simulink model "PP_vs_LQ_controllers_sim"  (R2019b)
settings: Solver=FixedStepAuto  StartTime=0.0  StopTime=10.0  FixedStep=0.002  RelTol=1e-3
values from neighbouring files (symbols this model uses):
  Ao = A-L*C    [StabilizationControl.m]
  Bo = [B,L]    [StabilizationControl.m]
  Co = eye(4)    [StabilizationControl.m]
  Klqi_int = Klqi(5)    [StabilizationControl.m]
  Klqi_state = Klqi(1:4)    [StabilizationControl.m]
  Kpp_int = Kpp_i(5)    [StabilizationControl.m]
  Kpp_state = Kpp_i(1:4)    [StabilizationControl.m]
undefined symbols (not defined in the file or in its folder): kalmf, Parameters
settings Model: Creator=Samsung  LastModifiedBy=Samsung

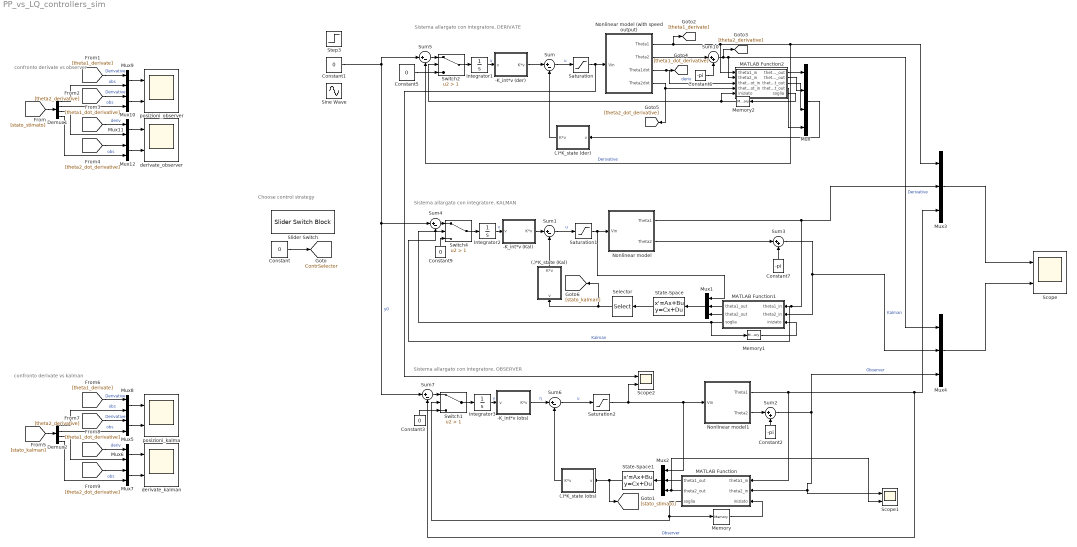
== system PP_vs_LQ_controllers_sim ==
  note: confronto derivate vs observer
  note: Choose control strategy
  note: Sistema allargato con integratore, DERIVATE
  note: Sistema allargato con integratore, KALMAN
  note: Sistema allargato con integratore, OBSERVER
  note: confronto derivate vs kalman
  (.)*K_state (Kal) : Subsystem
  "(.)*K_state (der) " : Subsystem
  (.)*K_state (obs) : Subsystem
  -K_int*v (Kal) : Subsystem
  -K_int*v (der) : Subsystem
  -K_int*v (obs) : Subsystem
  Constant{,1,3,5,9} (5 alike) : Constant  Value=0
  Constant2 : Constant  Value=-pi
  Constant6 : Constant  Value=-pi
  Constant7 : Constant  Value=-pi
  Demux1 : Demux
  Demux2 : Demux
  Integrator1 : Integrator
  Integrator2 : Integrator
  Integrator3 : Integrator
  MATLAB Function : MATLAB Function  TreatAsAtomicUnit=on
  MATLAB Function1 : MATLAB Function  TreatAsAtomicUnit=on
  MATLAB Function2 : MATLAB Function  TreatAsAtomicUnit=on
  Memory : Memory
  Memory1 : Memory  InitialCondition=false
  Memory2 : Memory
  Mux : Mux
  Mux{1..4} (4 alike) : Mux  Inputs=3
  Mux{5..12} (8 alike) : Mux  Inputs=2
  Nonlinear model : Subsystem
  Nonlinear model (with speed output) : Subsystem
  Nonlinear model1 : Subsystem
  Saturation : Saturate  UpperLimit=10  LowerLimit=-10
  Saturation1 : Saturate  UpperLimit=10  LowerLimit=-10
  Saturation2 : Saturate  UpperLimit=10  LowerLimit=-10
  Scope : Scope  NumInputPorts=2
  Scope1 : Scope  NumInputPorts=2
  Scope2 : Scope  NumInputPorts=2
  Selector : Selector  InputPortWidth=6  IndexOptions=Index vector (dialog)  Indices=[3,4,5,6]  OutputSizes=1
  Sine Wave : Sin  SampleTime=0
  Slider Switch : SliderSwitchBlock  LabelPosition=Hide
      settings: Values={{'PP', 'LQ'}, [0 1]}
  State-Space : StateSpace  A=kalmf.A  B=kalmf.B  C=kalmf.C  D=kalmf.D  InitialCondition=[0,0,0,0]
  State-Space1 : StateSpace  A=Ao  B=Bo  C=Co  D=zeros(4,3)  InitialCondition=[0,0,0,0]
  Step3 : Step  After=5  SampleTime=0
  Sum{,1,4..7} (6 alike) : Sum  Inputs=|+-
  Sum10 : Sum  Inputs=|++
  Sum2 : Sum  Inputs=|++
  Sum3 : Sum  Inputs=|++
  Switch1 : Switch  Criteria=u2 > Threshold  Threshold=1
  Switch2 : Switch  Criteria=u2 > Threshold  Threshold=1
  Switch4 : Switch  Criteria=u2 > Threshold  Threshold=1
  derivate_kalman : Scope  NumInputPorts=2
  "derivate_observer " : Scope  NumInputPorts=2
  posizioni_kalma : Scope  NumInputPorts=2
  posizioni_observer : Scope  NumInputPorts=2
  tag scope: ContrSelector=global
  wires:
  Sum2/1 -> Scope1/1, MATLAB Function/2(theta2_in), Mux4/3  "Observer"
  Saturation2/1 -> Scope2/2, Mux2/1, Nonlinear model1/1(Vin)
  Nonlinear model (with speed output)/1(Theta1) -> [theta1_derivate], MATLAB Function2/1(theta1_in), Mux3/1, Sum5/2  "Derivative"
  Mux2/1 -> State-Space1/1
  Nonlinear model (with speed output)/2(Theta2) -> Sum10/1
  State-Space/1 -> Selector/1
  Nonlinear model/1(Theta1) -> MATLAB Function1/1(theta1_in), Sum4/2, Mux3/2  "Kalman"
  "(.)*K_state (der) "/1(K*v) -> Sum/2
  Mux1/1 -> State-Space/1
  Sum3/1 -> MATLAB Function1/2(theta2_in), Mux4/2  "Kalman"
  Sum/1 -> Saturation/1  "u"
  Nonlinear model (with speed output)/3(Theta1dot) -> MATLAB Function2/3(theta1_dot_in), [theta1_dot_derivative]  "deriv"
  Nonlinear model1/1(Theta1) -> Sum7/2, Mux3/3, MATLAB Function/1(theta1_in)  "Observer"
  Sum6/1 -> Saturation2/1  "u"
  Nonlinear model (with speed output)/4(Theta2dot) -> [theta2_dot_derivative], MATLAB Function2/4(theta2_dot_in)
  Saturation1/1 -> Mux1/1, Nonlinear model/1(Vin)
  Constant7/1 -> Sum3/2
  -K_int*v (obs)/1(K*v) -> Sum6/1  "η"
  Constant6/1 -> Sum10/2
  Integrator1/1 -> -K_int*v (der)/1(v)  "v"
  Integrator3/1 -> -K_int*v (obs)/1(v)  "v"
  -K_int*v (der)/1(K*v) -> Sum/1
  (.)*K_state (Kal)/1(K*v) -> Sum1/2
  Sum10/1 -> MATLAB Function2/2(theta2_in), Mux4/1, [theta2_derivative]  "Derivative"
  Saturation/1 -> Scope2/1, Nonlinear model (with speed output)/1(Vin)
  Constant2/1 -> Sum2/2
  Nonlinear model/2(Theta2) -> Sum3/1
  Nonlinear model1/2(Theta2) -> Sum2/1
  Integrator2/1 -> -K_int*v (Kal)/1(v)  "v"
  Sum1/1 -> Saturation1/1  "u"
  -K_int*v (Kal)/1(K*v) -> Sum1/1
  Constant1/1 -> Sum7/1, Sum4/1, Sum5/1  "y0"
  Mux3/1 -> Scope/1
  Mux4/1 -> Scope/2
  Constant/1 -> [ContrSelector]
  Demux1/3 -> Mux11/2
  Mux9/1 -> posizioni_observer/1
  Mux11/1 -> "derivate_observer "/1
  Mux12/1 -> "derivate_observer "/2
  Demux1/2 -> Mux10/2  "obs"
  [theta2_derivative] -> Mux10/1  "Derivative"
  [theta1_derivate] -> Mux9/1  "Derivative"
  Mux10/1 -> posizioni_observer/2
  [theta1_dot_derivative] -> Mux11/1  "deriv"
  [theta2_dot_derivative] -> Mux12/1
  Demux1/1 -> Mux9/2  "obs"
  Demux1/4 -> Mux12/2  "obs"
  [stato_stimato] -> Demux1/1
  [theta2_dot_derivative] -> Mux7/1
  [stato_kalman] -> Demux2/1
  [theta1_derivate] -> Mux8/1  "Derivative"
  Demux2/4 -> Mux7/2  "obs"
  Mux5/1 -> posizioni_kalma/2
  Mux7/1 -> derivate_kalman/2
  Mux6/1 -> derivate_kalman/1
  Mux8/1 -> posizioni_kalma/1
  Demux2/3 -> Mux6/2
  Demux2/2 -> Mux5/2  "obs"
  [theta1_dot_derivative] -> Mux6/1  "deriv"
  Demux2/1 -> Mux8/2  "obs"
  [theta2_derivative] -> Mux5/1  "Derivative"
  MATLAB Function/1(theta1_out) -> Mux2/2
  MATLAB Function/2(theta2_out) -> Scope1/2, Mux2/3
  MATLAB Function/3(soglia) -> Switch1/2, Memory/1
  Memory/1 -> MATLAB Function/3(iniziato)
  MATLAB Function1/2(theta2_out) -> Mux1/3
  Memory1/1 -> MATLAB Function1/3(iniziato)
  MATLAB Function1/3(soglia) -> Memory1/1, Switch4/2
  MATLAB Function1/1(theta1_out) -> Mux1/2
  MATLAB Function2/2(theta2_out) -> Mux/2
  Memory2/1 -> MATLAB Function2/5(iniziato), Switch2/2
  MATLAB Function2/5(soglia) -> Memory2/1
  MATLAB Function2/1(theta1_out) -> Mux/1
  (.)*K_state (obs)/1(K*v) -> Sum6/2
  Sum7/1 -> Switch1/1
  Switch1/1 -> Integrator3/1
  Constant3/1 -> Switch1/3
  Sum5/1 -> Switch2/1
  Switch2/1 -> Integrator1/1
  Constant5/1 -> Switch2/3
  Mux/1 -> "(.)*K_state (der) "/1(v)
  Sum4/1 -> Switch4/1
  Switch4/1 -> Integrator2/1
  Constant9/1 -> Switch4/3
  Selector/1 -> (.)*K_state (Kal)/1(v), [stato_kalman]
  State-Space1/1 -> (.)*K_state (obs)/1(v), [stato_stimato]
  MATLAB Function2/3(theta1_dot_out) -> Mux/3
  MATLAB Function2/4(theta2_dot_out) -> Mux/4

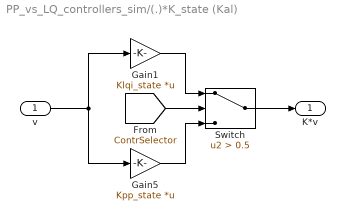
== system PP_vs_LQ_controllers_sim/(.)*K_state (Kal) ==
  v : Inport
  Gain1 : Gain  Gain=Klqi_state  Multiplication=Matrix(K*u)
  Gain5 : Gain  Gain=Kpp_state  Multiplication=Matrix(K*u)
  Switch : Switch  Criteria=u2 > Threshold  Threshold=0.5
  K*v : Outport
  wires:
  Switch/1 -> K*v/1
  Gain5/1 -> Switch/3
  Gain1/1 -> Switch/1
  v/1 -> Gain5/1, Gain1/1
  [ContrSelector] -> Switch/2

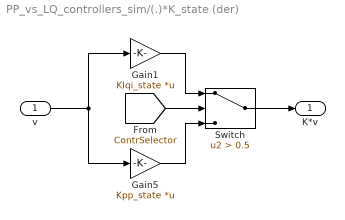
== system PP_vs_LQ_controllers_sim/(.)*K_state (der)  ==
  v : Inport
  Gain1 : Gain  Gain=Klqi_state  Multiplication=Matrix(K*u)
  Gain5 : Gain  Gain=Kpp_state  Multiplication=Matrix(K*u)
  Switch : Switch  Criteria=u2 > Threshold  Threshold=0.5
  K*v : Outport
  wires:
  Switch/1 -> K*v/1
  Gain5/1 -> Switch/3
  Gain1/1 -> Switch/1
  v/1 -> Gain5/1, Gain1/1
  [ContrSelector] -> Switch/2

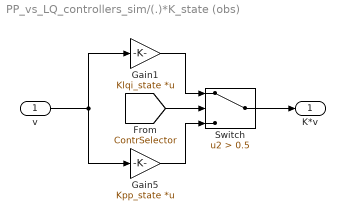
== system PP_vs_LQ_controllers_sim/(.)*K_state (obs) ==
  v : Inport
  Gain1 : Gain  Gain=Klqi_state  Multiplication=Matrix(K*u)
  Gain5 : Gain  Gain=Kpp_state  Multiplication=Matrix(K*u)
  Switch : Switch  Criteria=u2 > Threshold  Threshold=0.5
  K*v : Outport
  wires:
  Switch/1 -> K*v/1
  Gain5/1 -> Switch/3
  Gain1/1 -> Switch/1
  v/1 -> Gain5/1, Gain1/1
  [ContrSelector] -> Switch/2

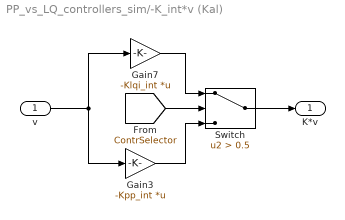
== system PP_vs_LQ_controllers_sim/-K_int*v (Kal) ==
  v : Inport
  Gain3 : Gain  Gain=-Kpp_int  Multiplication=Matrix(K*u)
  Gain7 : Gain  Gain=-Klqi_int  Multiplication=Matrix(K*u)
  Switch : Switch  Criteria=u2 > Threshold  Threshold=0.5
  K*v : Outport
  wires:
  Switch/1 -> K*v/1
  Gain3/1 -> Switch/3
  Gain7/1 -> Switch/1
  v/1 -> Gain3/1, Gain7/1
  [ContrSelector] -> Switch/2

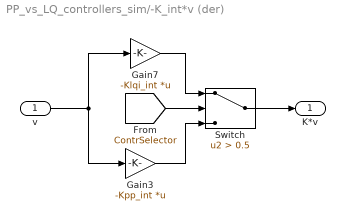
== system PP_vs_LQ_controllers_sim/-K_int*v (der) ==
  v : Inport
  Gain3 : Gain  Gain=-Kpp_int  Multiplication=Matrix(K*u)
  Gain7 : Gain  Gain=-Klqi_int  Multiplication=Matrix(K*u)
  Switch : Switch  Criteria=u2 > Threshold  Threshold=0.5
  K*v : Outport
  wires:
  Switch/1 -> K*v/1
  Gain3/1 -> Switch/3
  Gain7/1 -> Switch/1
  v/1 -> Gain3/1, Gain7/1
  [ContrSelector] -> Switch/2

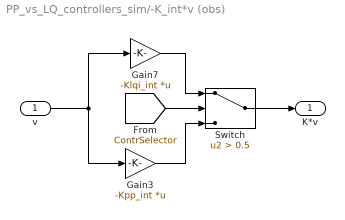
== system PP_vs_LQ_controllers_sim/-K_int*v (obs) ==
  v : Inport
  Gain3 : Gain  Gain=-Kpp_int  Multiplication=Matrix(K*u)
  Gain7 : Gain  Gain=-Klqi_int  Multiplication=Matrix(K*u)
  Switch : Switch  Criteria=u2 > Threshold  Threshold=0.5
  K*v : Outport
  wires:
  Switch/1 -> K*v/1
  Gain3/1 -> Switch/3
  Gain7/1 -> Switch/1
  v/1 -> Gain3/1, Gain7/1
  [ContrSelector] -> Switch/2

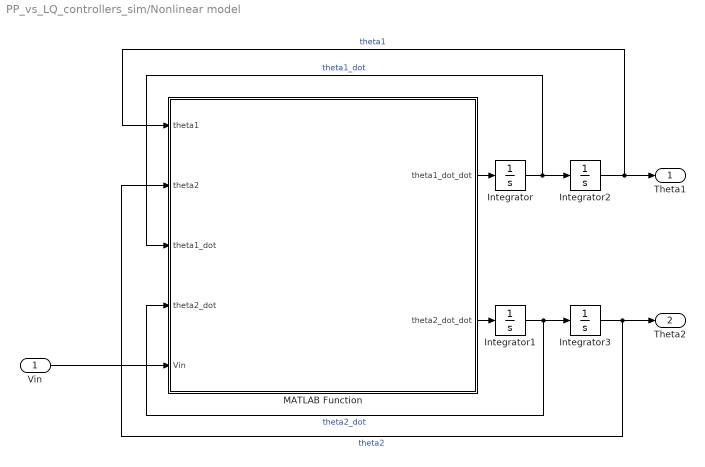
== system PP_vs_LQ_controllers_sim/Nonlinear model ==
  Vin : Inport
  Integrator : Integrator  InitialCondition=0.05
  Integrator1 : Integrator  InitialCondition=0.05
  Integrator2 : Integrator
  Integrator3 : Integrator  InitialCondition=pi
  MATLAB Function : MATLAB Function  TreatAsAtomicUnit=on  mask{Pars=Parameters}
      mask prompts: Pars "Struct containing model parameters"
  Theta1 : Outport
  Theta2 : Outport  Port=2
  wires:
  Integrator/1 -> MATLAB Function/3(theta1_dot), Integrator2/1  "theta1_dot"
  Integrator1/1 -> MATLAB Function/4(theta2_dot), Integrator3/1  "theta2_dot"
  MATLAB Function/1(theta1_dot_dot) -> Integrator/1
  Integrator3/1 -> Theta2/1, MATLAB Function/2(theta2)  "theta2"
  MATLAB Function/2(theta2_dot_dot) -> Integrator1/1
  Integrator2/1 -> MATLAB Function/1(theta1), Theta1/1  "theta1"
  Vin/1 -> MATLAB Function/5(Vin)

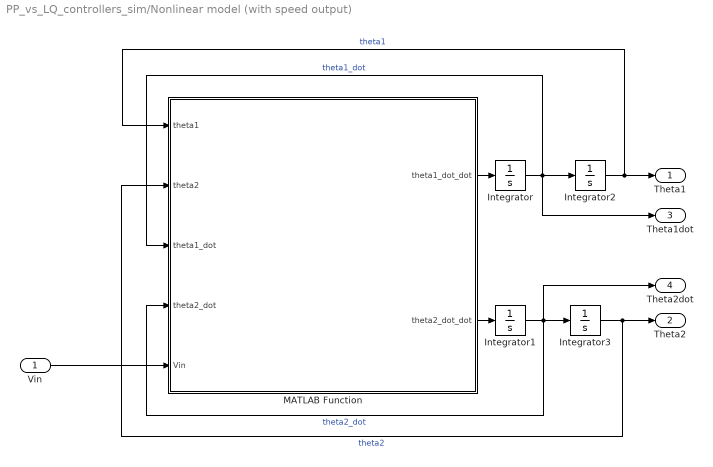
== system PP_vs_LQ_controllers_sim/Nonlinear model (with speed output) ==
  Vin : Inport
  Integrator : Integrator  InitialCondition=0.05
  Integrator1 : Integrator  InitialCondition=0.05
  Integrator2 : Integrator
  Integrator3 : Integrator  InitialCondition=pi
  MATLAB Function : MATLAB Function  TreatAsAtomicUnit=on  mask{Pars=Parameters}
      mask prompts: Pars "Struct containing model parameters"
  Theta1 : Outport
  Theta2 : Outport  Port=2
  Theta1dot : Outport  Port=3
  Theta2dot : Outport  Port=4
  wires:
  Integrator/1 -> Theta1dot/1, MATLAB Function/3(theta1_dot), Integrator2/1  "theta1_dot"
  Integrator1/1 -> Theta2dot/1, MATLAB Function/4(theta2_dot), Integrator3/1  "theta2_dot"
  MATLAB Function/1(theta1_dot_dot) -> Integrator/1
  Integrator3/1 -> Theta2/1, MATLAB Function/2(theta2)  "theta2"
  MATLAB Function/2(theta2_dot_dot) -> Integrator1/1
  Integrator2/1 -> MATLAB Function/1(theta1), Theta1/1  "theta1"
  Vin/1 -> MATLAB Function/5(Vin)

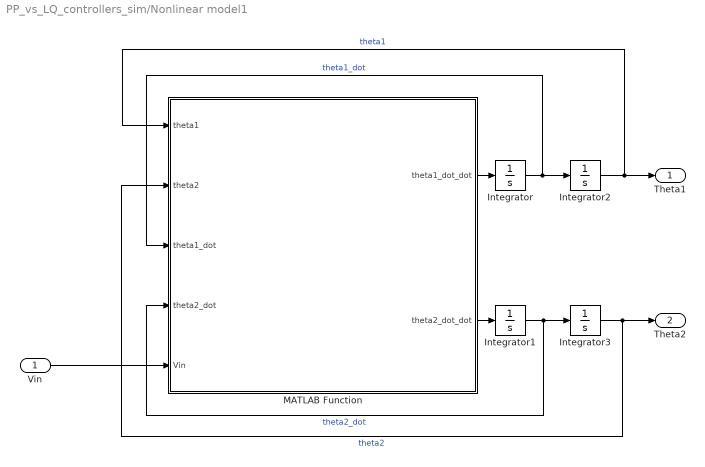
== system PP_vs_LQ_controllers_sim/Nonlinear model1 ==
  Vin : Inport
  Integrator : Integrator  InitialCondition=0.05
  Integrator1 : Integrator  InitialCondition=0.05
  Integrator2 : Integrator
  Integrator3 : Integrator  InitialCondition=pi
  MATLAB Function : MATLAB Function  TreatAsAtomicUnit=on  mask{Pars=Parameters}
      mask prompts: Pars "Struct containing model parameters"
  Theta1 : Outport
  Theta2 : Outport  Port=2
  wires:
  Integrator/1 -> MATLAB Function/3(theta1_dot), Integrator2/1  "theta1_dot"
  Integrator1/1 -> MATLAB Function/4(theta2_dot), Integrator3/1  "theta2_dot"
  MATLAB Function/1(theta1_dot_dot) -> Integrator/1
  Integrator3/1 -> Theta2/1, MATLAB Function/2(theta2)  "theta2"
  MATLAB Function/2(theta2_dot_dot) -> Integrator1/1
  Integrator2/1 -> MATLAB Function/1(theta1), Theta1/1  "theta1"
  Vin/1 -> MATLAB Function/5(Vin)

== matlab function PP_vs_LQ_controllers_sim/Nonlinear model1/MATLAB Function ==
  data: theta1 input; theta1_dot_dot output; theta2 input; theta1_dot input; theta2_dot input; Vin input; theta2_dot_dot output; Pars parameter
function [theta1_dot_dot,theta2_dot_dot] = fcn(theta1, theta2, theta1_dot, theta2_dot,Vin, Pars)

   k1 = Pars.Jeq + Pars.m2*(Pars.l1^2 + Pars.x2^2*sin(theta2)^2);
   k2 = Pars.m2*Pars.l1*Pars.x2*cos(theta2);
   k3 = 2*Pars.m2*Pars.x2^2*sin(theta2)*cos(theta2)*theta1_dot*theta2_dot - Pars.m2*Pars.l1*Pars.x2*sin(theta2)*theta2_dot^2 +Pars.Ks*theta1 - Pars.Km/Pars.Rm*Vin + (Pars.Km^2)/Pars.Rm*theta1_dot + Pars.Kf1*theta1_dot;
   k4 = Pars.m2*Pars.l1*Pars.x2*cos(theta2);
   k5 = Pars.m2*Pars.x2^2 + Pars.I2;
   k6 = - Pars.m2*Pars.x2^2*sin(theta2)*cos(theta2)*theta1_dot^2 + Pars.m2*Pars.g*Pars.x2*sin(theta2) + Pars.Kf2*theta2_dot;


theta1_dot_dot = (k2*k6 - k3*k5)/(k1*k5 - k2*k4);
theta2_dot_dot = -(k1*k6 - k3*k4)/(k1*k5 - k2*k4);

== matlab function PP_vs_LQ_controllers_sim/Nonlinear model/MATLAB Function ==
  data: theta1 input; theta1_dot_dot output; theta2 input; theta1_dot input; theta2_dot input; Vin input; theta2_dot_dot output; Pars parameter
function [theta1_dot_dot,theta2_dot_dot] = fcn(theta1, theta2, theta1_dot, theta2_dot,Vin, Pars)

   k1 = Pars.Jeq + Pars.m2*(Pars.l1^2 + Pars.x2^2*sin(theta2)^2);
   k2 = Pars.m2*Pars.l1*Pars.x2*cos(theta2);
   k3 = 2*Pars.m2*Pars.x2^2*sin(theta2)*cos(theta2)*theta1_dot*theta2_dot - Pars.m2*Pars.l1*Pars.x2*sin(theta2)*theta2_dot^2 +Pars.Ks*theta1 - Pars.Km/Pars.Rm*Vin + (Pars.Km^2)/Pars.Rm*theta1_dot + Pars.Kf1*theta1_dot;
   k4 = Pars.m2*Pars.l1*Pars.x2*cos(theta2);
   k5 = Pars.m2*Pars.x2^2 + Pars.I2;
   k6 = - Pars.m2*Pars.x2^2*sin(theta2)*cos(theta2)*theta1_dot^2 + Pars.m2*Pars.g*Pars.x2*sin(theta2) + Pars.Kf2*theta2_dot;


theta1_dot_dot = (k2*k6 - k3*k5)/(k1*k5 - k2*k4);
theta2_dot_dot = -(k1*k6 - k3*k4)/(k1*k5 - k2*k4);

== matlab function PP_vs_LQ_controllers_sim/MATLAB Function ==
  data: theta1_in input; theta1_out output; theta2_out output; theta2_in input; iniziato input double; soglia output double
function [theta1_out, theta2_out, soglia] = fcn(theta1_in, theta2_in, iniziato)
if theta2_in >= 0.01
    theta1_out = theta1_in;
    theta2_out = theta2_in;
    soglia = 2; 
elseif iniziato >1
    theta1_out = theta1_in;
    theta2_out = theta2_in;
    soglia = 2;
else
    soglia = 0;
    theta1_out = 0;
    theta2_out = 0;
end
end

== matlab function PP_vs_LQ_controllers_sim/Nonlinear model (with speed output)/MATLAB Function ==
  data: theta1 input; theta1_dot_dot output; theta2 input; theta1_dot input; theta2_dot input; Vin input; theta2_dot_dot output; Pars parameter
function [theta1_dot_dot,theta2_dot_dot] = fcn(theta1, theta2, theta1_dot, theta2_dot,Vin, Pars)

   k1 = Pars.Jeq + Pars.m2*(Pars.l1^2 + Pars.x2^2*sin(theta2)^2);
   k2 = Pars.m2*Pars.l1*Pars.x2*cos(theta2);
   k3 = 2*Pars.m2*Pars.x2^2*sin(theta2)*cos(theta2)*theta1_dot*theta2_dot - Pars.m2*Pars.l1*Pars.x2*sin(theta2)*theta2_dot^2 +Pars.Ks*theta1 - Pars.Km/Pars.Rm*Vin + (Pars.Km^2)/Pars.Rm*theta1_dot + Pars.Kf1*theta1_dot;
   k4 = Pars.m2*Pars.l1*Pars.x2*cos(theta2);
   k5 = Pars.m2*Pars.x2^2 + Pars.I2;
   k6 = - Pars.m2*Pars.x2^2*sin(theta2)*cos(theta2)*theta1_dot^2 + Pars.m2*Pars.g*Pars.x2*sin(theta2) + Pars.Kf2*theta2_dot;


theta1_dot_dot = (k2*k6 - k3*k5)/(k1*k5 - k2*k4);
theta2_dot_dot = -(k1*k6 - k3*k4)/(k1*k5 - k2*k4);

== matlab function PP_vs_LQ_controllers_sim/MATLAB Function1 ==
  data: theta1_in input; theta1_out output; theta2_in input; iniziato input double; theta2_out output; soglia output
function [theta1_out, theta2_out, soglia] = fcn(theta1_in, theta2_in, iniziato)
if theta2_in >= 0.01
    theta1_out = theta1_in;
    theta2_out = theta2_in;
    soglia = 2; 
elseif iniziato >1
    theta1_out = theta1_in;
    theta2_out = theta2_in;
    soglia = 2;
else
    soglia = 0;
    theta1_out = 0;
    theta2_out = 0;
end
% soglia = 2;s
% theta1_out = theta1_in;
% theta2_out = theta2_in;
end

== matlab function PP_vs_LQ_controllers_sim/MATLAB Function2 ==
  data: theta1_in input; theta1_out output; theta2_in input; theta1_dot_in input; theta2_dot_in input; iniziato input double; theta2_out output; theta1_dot_out output; theta2_dot_out output; soglia output double
function [theta1_out, theta2_out, theta1_dot_out, theta2_dot_out, soglia] = fcn(theta1_in, theta2_in, theta1_dot_in, theta2_dot_in, iniziato)
if theta2_in >= 0.01
    theta1_out = theta1_in;
    theta2_out = theta2_in;
    theta1_dot_out = theta1_dot_in;
    theta2_dot_out = theta2_dot_in;
    soglia = 2; 
elseif iniziato >1
    theta1_out = theta1_in;
    theta2_out = theta2_in;
    theta1_dot_out = theta1_dot_in;
    theta2_dot_out = theta2_dot_in;
    soglia = 2;
else
    soglia = 0;
    theta1_out = 0;
    theta2_out = 0;
    theta1_dot_out = 0;
    theta2_dot_out = 0;
end
% soglia = 2;
% theta1_out = theta1_in;
% theta2_out = theta2_in;
end
